simulink model "movingAverage"  (R2017a)
settings: Solver=FixedStepDiscrete  StartTime=0.0  StopTime=100  FixedStep=0.01  RelTol=1e-3
undefined symbols (not defined in the file): f, mdl_T_sample
libraries: simulink x1, dspindex x1
settings Model: Creator=kando  LastModifiedBy=kando

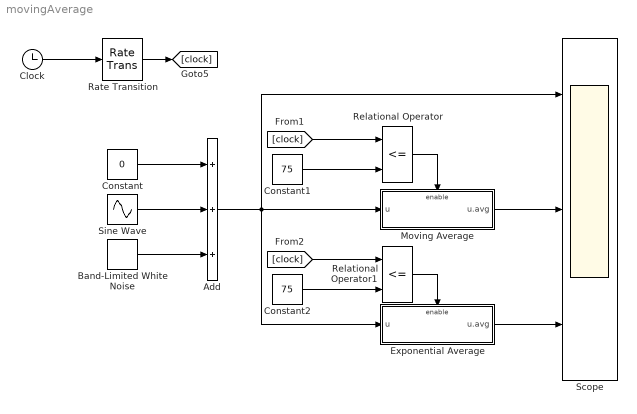
== system movingAverage ==
  Add : Sum  Inputs=+++
  Band-Limited White Noise : simulink/Sources/Band-Limited White Noise  Cov=[0.0001]  Ts=0.01  seed=[23341]
  Clock : Clock
      settings: Decimation=round( 1 / mdl_T_sample )
  Constant : Constant  Value=0  SampleTime=0.01
  Constant1 : Constant  Value=75  SampleTime=0.01
  Constant2 : Constant  Value=75  SampleTime=0.01
  Exponential Average : Subsystem  mask{alpha=1-exp(-2*pi*10*0.01)}
  Moving Average : Subsystem  mask{N=100}
  Rate Transition : RateTransition  OutPortSampleTime=mdl_T_sample
  Relational Operator : RelationalOperator  Operator=<=  OutDataTypeStr=boolean  RndMeth=Simplest
  Relational Operator1 : RelationalOperator  Operator=<=  OutDataTypeStr=boolean  RndMeth=Simplest
  Scope : Scope  NumInputPorts=3
  Sine Wave : Sin  Amplitude=0.05  SampleTime=0.01
  wires:
  Band-Limited White Noise/1 -> Add/3
  Sine Wave/1 -> Add/2
  Constant/1 -> Add/1
  Moving Average/1(u.avg) -> Scope/2
  Exponential Average/1(u.avg) -> Scope/3
  Add/1 -> Moving Average/1(u), Exponential Average/1(u), Scope/1
  Clock/1 -> Rate Transition/1
  Rate Transition/1 -> [clock]
  [clock] -> Relational Operator/1
  [clock] -> Relational Operator1/1
  Constant1/1 -> Relational Operator/2
  Constant2/1 -> Relational Operator1/2
  Relational Operator1/1 -> Exponential Average/Enable
  Relational Operator/1 -> Moving Average/Enable

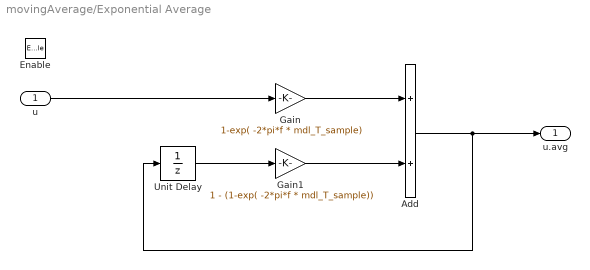
== system movingAverage/Exponential Average ==
  u : Inport
  Enable : EnablePort
  Add : Sum
  Gain : Gain  Gain=1-exp( -2*pi*f * mdl_T_sample)
      settings: AttributesFormatString=%<Gain>
  Gain1 : Gain  Gain=1 - (1-exp( -2*pi*f * mdl_T_sample))
      settings: AttributesFormatString=%<Gain>
  Unit Delay : UnitDelay  SampleTime=-1
  u.avg : Outport
  wires:
  Gain/1 -> Add/1
  u/1 -> Gain/1
  Unit Delay/1 -> Gain1/1
  Gain1/1 -> Add/2
  Add/1 -> Unit Delay/1, u.avg/1

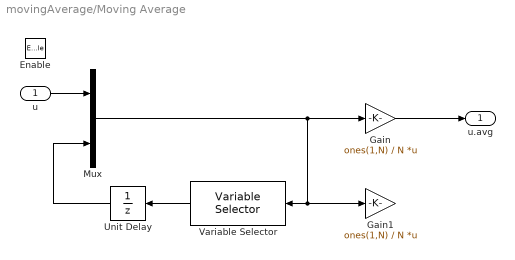
== system movingAverage/Moving Average ==
  u : Inport
  Enable : EnablePort
  Gain : Gain  Gain=ones(1,N) / N  Multiplication=Matrix(K*u)
      settings: AttributesFormatString=%<Gain>
  Gain1 : Gain  Gain=ones(1,N) / N  Multiplication=Matrix(K*u)
      settings: AttributesFormatString=%<Gain>
  Mux : Mux  Inputs=2
  Unit Delay : UnitDelay  InitialCondition=zeros(N-1,1)  SampleTime=-1
  Variable Selector : dspindex/Variable Selector  NumInputs=1  rowsOrCols=Rows  IdxMode=Fixed  Elements=[ 1 : (N-1) ]  ZerOneIdxMode=One-based  errmode=Clip Index  FillMode=on  FillValues=0
  u.avg : Outport
  wires:
  Mux/1 -> Gain1/1, Variable Selector/1, Gain/1
  Variable Selector/1 -> Unit Delay/1
  Gain/1 -> u.avg/1
  Unit Delay/1 -> Mux/2
  u/1 -> Mux/1
